simulink model "HEV_powersplit_adapted"  (R2026a)
settings: Solver=VariableStepAuto  StopTime=DriveCycles(Drive_Cycle_Num).time(end)  FixedStep=Ts  AbsTol=1e-3  EnableMultiTasking=on
PreLoadFcn:
  | mdlDir = fileparts(get_param(bdroot,'FileName'));
  | if exist(mdlDir,'dir'), addpath(genpath(mdlDir)); end;
  | HEV_Model_HomeDir = mdlDir;
  | decimation = 1;
  | HEV_Model_PARAM;
  | HEV_SeriesParallel_param_detailed;
StartFcn:
  | tic;
StopFcn:
  | Elapsed_Sim_Time = toc;
undefined symbols (not defined in the file): AH, AH0, Drive_Cycle_Num, HEV_Param, Ld, Lq, p, psim, System, Ts, Vbat, VDC_VECT
libraries: fl_lib x70, nesl_utility x54, ee_lib x10, sdl_lib x6, eeTransforms x4, eePmsmCurrentController x2, eeGeneralControl x2, eePmsmCurrentReferenceGen x2, eePwmGeneratorTwoLevel x2, batteryecm_lib x1, Capacitors_lib x1, eePmsmTorqueEstimator x1
(part 1 of 3)
CloseFcn:
  | try,close(h1_HEV_powersplit_adapted),end
  | try,close(h2_HEV_powersplit_adapted),end
  | try,close(h3_HEV_powersplit_adapted),end
  | try,close(h4_hev_powersplit_adapted_pct),end
  | clear h1_HEV_powersplit_adapted h2_HEV_powersplit_adapted h3_HEV_powersplit_adapted h4_hev_powersplit_adapted_pct
  | clear simlog_HEV_powersplit_adapted logsout_HEV_powersplit_adapted Elapsed_Sim_Time
  | 
  | try,close(h1_IPMSMSeriesParallelHEV),end
  | clear h1_IPMSMSeriesParallelHEV
  | 
  | clear simlog_IPMSMSeriesParallelHEV
  | clear logsout_IPMSMSeriesParallelHEV
  | 
  | clear PmaxEM TmaxEM p psim Ld Lq L0 Rs Jm Cdc Vnom
  | clear Q Vbat Ri AH V1 AH1 SOC0 AH0
  | clear TmaxICE PmaxICE Km Tm
  | clear Ts fsw Tsi Tso Tsd Kp_id Ki_id Kp_iq Ki_iq
  | clear numd_id dend_id numd_iq dend_iq
  | clear Kp_ice Ki_ice Kp_omega Ki_omega numd_omega dend_omega
  | clear ID_MAP IQ_MAP RPM_VECT TQ_VECT VDC_VECT
  | clear Mv g rho_a AL Cd cr1 cr2 Rw ratio i_t
Description:
  | IPMSM Torque Control in a Series-Parallel HEV
  | Copyright 2025 The MathWorks, Inc.
settings Model: NumberOfSteps=100  Creator=The MathWorks, Inc.  LastModifiedBy=gusta
settings DataIOCC: MaxDataPoints=310000  SignalLoggingName=logsout_HEV_powersplit_adapted
settings OptimizationCC: OptimizeBlockIOStorage=off  OptimizeDataStoreBuffers=off  BusAssignmentInplaceUpdate=off
settings DebuggingCC: UnderspecifiedInitializationDetection=Classic  MaxConsecutiveZCsMsg=none  MaskedZcDiagnostic=none  IgnoredZcDiagnostic=none  ParameterPrecisionLossMsg=none
settings RTWCC: GenerateReport=on  BuildConfiguration=Debug  LaunchReport=on
settings CodeAppCC: MATLABSourceComments=on  EnableCustomComments=on
settings GRTTargetCC: MultiInstanceErrorCode=Warning  CombineSignalStateStructs=on  SupportVariableSizeSignals=on
settings SimscapeCC: SimscapeNormalizeSystem=off  SimscapeNominalValues="[{\"value\":\"1\",\"unit\":\"A\"},{\"value\":\"1\",\"unit\":\"bar\"},{\"value\":\"1\",\"unit\":\"cm^2\"},{\"value\":\"1\",\"unit\":\"cm^3/s\"},{\"value\":\"1\",\"unit\":\"kJ/kg\"},{\"value\":\"1\",\"unit\":\"kW\"},{\"value\":\"1\",\"unit\":\"l\"},{\"value\":\"1\",\"unit\":\"N\"},{\"value\":\"1\",\"unit\":\"N*m\"},{\"value\":\"1\",\"unit\":\"V\"}]"  SimscapeLogSimulationStatistics=on  SimscapeLogName=simlog_HEV_powersplit_adapted  SimscapeLogDataHistory=310000.0

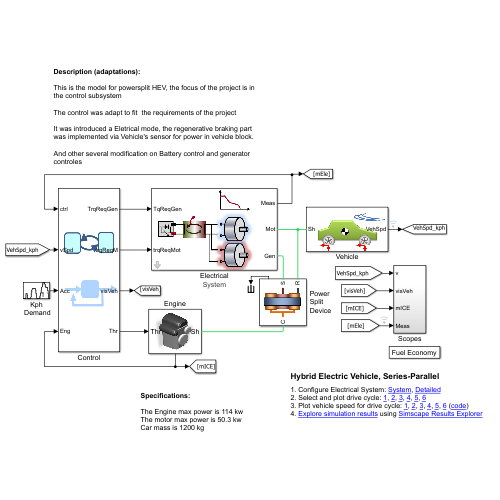
[thumbnail: Simulink's stored preview of the top-level diagram]
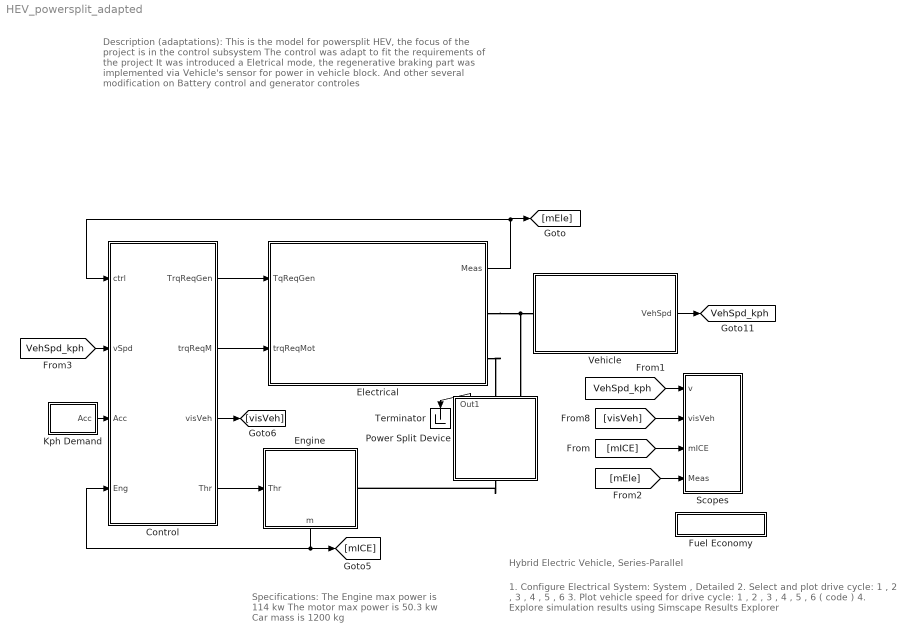
== system HEV_powersplit_adapted ==
  note: Description (adaptations):
      |
      | This is the model for powersplit HEV, the focus of the project is in the control subsystem
      |
      | The control was adapt to fit the requirements of the project
      |
      | It was introduced a Eletrical mode, the regenerative braking part was implemented via Vehicle's sensor for power in vehicle block.
      |
      | And other several modification on Battery control and generator controles
  note: Specifications:
      |
      | The Engine max power is 114 kw
      | The motor max power is 50.3 kw
      | Car mass is 1200 kg
  note: Hybrid Electric Vehicle, Series-Parallel
  note: 1. Configure Electrical System: System , Detailed
      | 2. Select and plot drive cycle: 1 , 2 , 3 , 4 , 5 , 6
      | 3. Plot vehicle speed for drive cycle: 1 , 2 , 3 , 4 , 5 , 6 ( code )
      | 4. Explore simulation results using Simscape Results Explorer
  Control : Subsystem
      mask Display: image('HEV_Control_IMAGE.jpg')
  Electrical : Subsystem  mask{popup_machModelType=System}
      mask prompts: popup_machModelType "Machine Model Type"
      settings: AttributesFormatString=%<popup_machModelType>
      mask TypeOptions popup_machModelType: Generator/popup_modelType | Motor/popup_modelType
      mask Display:
      | bh = gcb;
      | machType = get_param(bh, 'popup_machModelType');
      | if(strcmp(machType,'Detailed'))
      |     image('HEV_Electrical_Detailed_Generic_IMAGE.jpg');
      | else
      |     image('HEV_Electrical_SystemLevel_Generic_IMAGE.jpg');
      | end
  Engine : Subsystem
      settings: PortSchema="{\"entries\":[{\"content\":{\"sides\":[{\"content\":{\"connectorIds\":[\"In1\"]},\"type\":\"ConnectorPlacement.EquallySpacedRectSide\",\"uuid\":\"790115e8-146c-4b4e-bf41-f4d786beb81e\"},{\"content\":{\"connectorIds\":[\"RConn1\"],\"side\":\"RIGHT\"},\"type\":\"ConnectorPlacement.EquallySpacedRectSide\",\"uuid\":\"b4f77556-b395-4615-ac3d-7576af564f11\"},{\"content\":{\"side\":\"TOP\"},\"type\":\"ConnectorPlacement.EquallySpacedRectSide\",\"uuid\":\"44f1e3da-b746-41cb-9fdb-85dae22187d3\"},{\"content\":{\"connectorIds\":[\"Out1\"],\"side\":\"BOTTOM\"},\"type\":\"ConnectorPlacement.EquallySpacedRectSide\",\"uuid\":\"b1d76e0d-1938-4db2-9fd9-287b303ac6ee\"}]},\"type\":\"ConnectorPlacement.EquallySpacedConnector\",\"uuid\":\"a06ee764-44f8-463f-a9be-99a8119a4dd7\"}],\"packageUris\":[\"http://schema.mathworks.com/mf0/Connector/R2020b\"],\"version\":\"1.0\"}"
      mask Display:
      | image('HEV_Engine_IMAGE.jpg');
      | port_label('input',1,'Thr');
      | port_label('RConn',1,'Sh');
  Fuel Economy : Subsystem  mask(Data Acquisition){}
      mask Display: disp('Fuel Economy');
  Kph Demand : Subsystem
      mask Display:
      | %if(evalin('base','Drive_Cycle_Num')<5)
      | plotstr=['UrbanCycle' evalin('base','num2str(Drive_Cycle_Num)')];
      | plot(evalin('base',[plotstr '.time']),evalin('base',[plotstr '.SpdKph']));
      | text(evalin('base',['0.7*max(' plotstr '.time)']),evalin('base',['0.25*max(' plotstr '.SpdKph)']),evalin('base','num2str(Drive_Cycle_Num)'));
      | %end
  Power Split Device : Subsystem
      mask Display:
      | image('HEV_Planetary_Gear_IMAGE.jpg');
      | color('black');
  Scopes : Subsystem
  Terminator : Terminator
  Vehicle : Subsystem  VariantControl=Full
      mask Display: image(imread('HEV_Vehicle_Dynamics_Full_IMAGE.jpg'));
  tag scope: VehSpd_kph=global
  wires:
  Kph Demand/1(Acc) -> Control/3(Acc)
  Control/3(visVeh) -> [visVeh]
  Vehicle/1(VehSpd) -> [VehSpd_kph]
  [visVeh] -> Scopes/2(visVeh)
  [VehSpd_kph] -> Scopes/1(v)
  Control/4(Thr) -> Engine/1(Thr)
  Engine/1(m) -> [mICE], Control/4(Eng)
  Control/1(TrqReqGen) -> Electrical/1(TqReqGen)
  Control/2(trqReqM) -> Electrical/2(trqReqMot)
  Electrical/1(Meas) -> Control/1(ctrl), [mEle]
  [mICE] -> Scopes/3(mICE)
  [mEle] -> Scopes/4(Meas)
  [VehSpd_kph] -> Control/2(vSpd)
  Power Split Device/1(Out1) -> Terminator/1
  connections:
  Electrical/RConn1 -- Power Split Device/RConn2 -- Vehicle/LConn1
  Power Split Device/LConn1 -- Engine/RConn1
  Electrical/RConn2 -- Power Split Device/RConn1

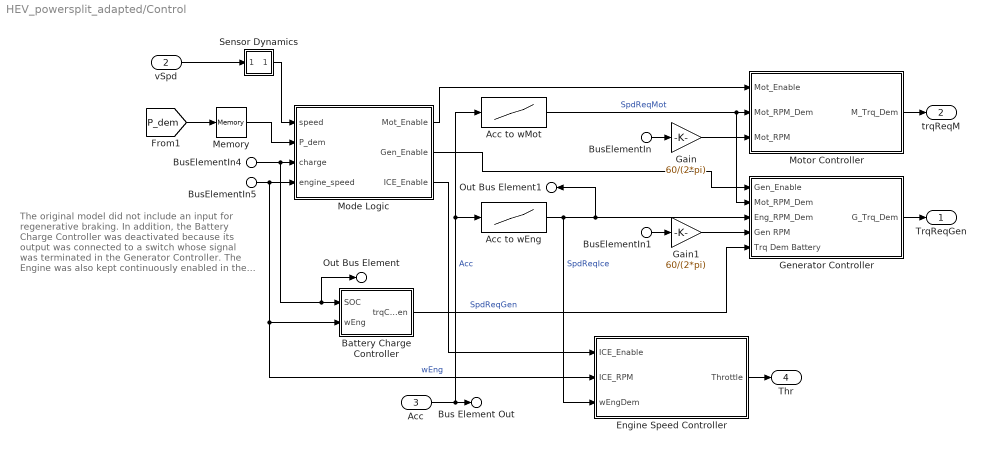
== system HEV_powersplit_adapted/Control ==
  note: The original model did not include an input for regenerative braking. In addition, the Battery Charge Controller was deactivated because its output was connected to a switch whose signal was terminated in the Generator Controller. The Engine was also kept continuously enabled in the Engine Speed Controller, bypassing the mode logic signal.
      | In addition, the sensor signal from the Vehicle block, P_dem , is now used as the power demand input to evaluate all mode transitions, including Regenerative Braking.
  BusElementIn4 : Inport  PortName=ctrl  Element=Batt.SOC
  BusElementIn : Inport  PortName=ctrl  Element=MotCtrl.w
  BusElementIn1 : Inport  PortName=ctrl  Element=GenCtrl.w
  vSpd : Inport  Port=2
  Acc : Inport  Port=3
  BusElementIn5 : Inport  Port=4  PortName=Eng  Element=wEng
  Acc to wEng : Lookup_n-D  NumberOfTableDimensions=1  BreakpointsForDimension1=[0 0.9 0.95 1]  Table=[800 5000 6000 6000]  InternalRulePriority=Speed  RndMeth=Simplest
  Acc to wMot : Lookup_n-D  NumberOfTableDimensions=1  BreakpointsForDimension1=[0 1 1.2]  Table=[0 6000 6000]  InternalRulePriority=Speed  RndMeth=Simplest
  Battery Charge Controller : Subsystem
  Engine Speed Controller : Subsystem
  Gain : Gain  Gain=60/(2*pi)
  Gain1 : Gain  Gain=60/(2*pi)
  Generator Controller : Subsystem
  Memory : Memory
  Mode Logic : Stateflow chart  TreatAsAtomicUnit=on
  Motor Controller : Subsystem
  Sensor Dynamics : Subsystem  mask(First-order lag supporting vector signals){b=HEV_Param.ICE.sensor_time_constant, x_initial=0}
      mask prompts: b "Filter time constant"; x_initial "Initial output"
      mask help: Models a lag of the form 1/(b*s+1) where s is the Laplace operator.
  TrqReqGen : Outport  VectorParamsAs1DForOutWhenUnconnected=off
  trqReqM : Outport  Port=2  VectorParamsAs1DForOutWhenUnconnected=off
  Bus Element Out : Outport  Port=3  PortName=visVeh  Element=Acc
  Out Bus Element : Outport  Port=3  PortName=visVeh  Element=SOC
  Out Bus Element1 : Outport  Port=3  PortName=visVeh  Element=wICEreq
  Thr : Outport  Port=4  VectorParamsAs1DForOutWhenUnconnected=off
  wires:
  Acc/1 -> Acc to wMot/1, Acc to wEng/1, Bus Element Out/1  "Acc"
  Mode Logic/2(Gen_Enable) -> Generator Controller/1(Gen_Enable)
  Generator Controller/1(G_Trq_Dem) -> TrqReqGen/1
  Mode Logic/1(Mot_Enable) -> Motor Controller/1(Mot_Enable)
  BusElementIn/1 -> Gain/1
  Motor Controller/1(M_Trq_Dem) -> trqReqM/1
  Mode Logic/3(ICE_Enable) -> Engine Speed Controller/1(ICE_Enable)
  Engine Speed Controller/1(Throttle) -> Thr/1
  Battery Charge Controller/1(trqCmdGen) -> Generator Controller/5(Trq Dem Battery)  "SpdReqGen"
  Acc to wEng/1 -> Generator Controller/3(Eng_RPM_Dem), Out Bus Element1/1, Engine Speed Controller/3(wEngDem)  "SpdReqIce"
  Acc to wMot/1 -> Generator Controller/2(Mot_RPM_Dem), Motor Controller/2(Mot_RPM_Dem)  "SpdReqMot"
  BusElementIn1/1 -> Gain1/1
  BusElementIn4/1 -> Out Bus Element/1, Battery Charge Controller/1(SOC), Mode Logic/3(charge)
  vSpd/1 -> Sensor Dynamics/1(In)
  BusElementIn5/1 -> Engine Speed Controller/2(ICE_RPM), Battery Charge Controller/2(wEng), Mode Logic/4(engine_speed)  "wEng"
  Sensor Dynamics/1(Out) -> Mode Logic/1(speed)
  Gain/1 -> Motor Controller/3(Mot_RPM)
  Gain1/1 -> Generator Controller/4(Gen RPM)
  [P_dem] -> Memory/1
  Memory/1 -> Mode Logic/2(P_dem)

== system HEV_powersplit_adapted/Electrical ==
  TqReqGen : Inport
  trqReqMot : Inport  Port=2
  DC-DC Converter : Subsystem
      mask Display:
      | patch([-0.9 -1 -1 0.9 1 1 -0.9],[-1 -1 -0.9 1 1 0.9 -1],[0 0 0])
      | 
      | patch([-0.8 -0.1 -0.1 -0.8],[0.85 0.85 0.75 0.75],[0 0 0])
      | patch([-0.8 -0.55 -0.55 -0.8],[0.65 0.65 0.55 0.55],[0 0 0])
      | patch([-0.35 -0.1 -0.1 -0.35],[0.65 0.65 0.55 0.55],[0 0 0])
      | 
      | patch([-0.8 -0.1 -0.1 -0.8]*-1,[0.65 0.65 0.55 0.55]*-1,[0 0 0])
      | patch([-0.8 -0.55 -0.55 -0.8]*-1,[0.85 0.85 0.75 0.75]*-1,[0 0 0])
      | patch([-0.35 -0.1 -0.1 -0.35]*-1,[0.85 0.85 0.75 0.75]*-1,[0 0 0])
  ERef : fl_lib/Electrical/Electrical Elements/Electrical Reference
  Electrical Reference : fl_lib/Electrical/Electrical Elements/Electrical Reference
  Generator : Subsystem  Variant=on  VariantControlMode=label  VariantControl=Generator  LabelModeActiveChoice=System  mask{popup_modelType=System}
      mask prompts: popup_modelType "Model Type"
      mask init:
      | bh = gcb;
      | set_param(bh,'LabelModeActiveChoice',get_param(bh,'popup_modelType'));
      mask TypeOptions popup_modelType: System | Detailed
  Generic : Subsystem  VariantControl=Generic
      mask Display: image('HEV_Battery_Custom_IMAGE.jpg')
  Motor : Subsystem  Variant=on  VariantControlMode=label  VariantControl=Motor  LabelModeActiveChoice=System  mask{popup_modelType=System}
      mask prompts: popup_modelType "Model Type"
      mask init:
      | bh = gcb;
      | set_param(bh,'LabelModeActiveChoice',get_param(bh,'popup_modelType'));
      mask TypeOptions popup_modelType: System | Detailed
  Solver Configuration : nesl_utility/Solver Configuration  PhysicalDomain=network_engine_domain  SubClassName=solver  LeftPortType=input  RightPortType=generic  Tones=[]  Harmonics=[]  SimulateNoise=off  Profile=off  UseLocalSampling=off  EnableSwitchedLinearOptims=on  FrequencyDomain=off  UseCCode=off  RelTol=0.001  AbsTol=1e-06  MinStep=1e-09  ToWorkspace=off  RevertToSquareIcSolve=off  NumHomotopyIterations=100  PhasorMode=off  PhasorModeNumHarmonics=1  ConsistencySolver=NEWTON_FTOL  CanonicalOrdering=UNORDERED  OptimizeIntermediates=UNOPTIMIZED  IndexReductionMethod=DerivativeReplacement  DoDC=off  ResidualTolerance=1e-9  ConsistencyTolSource=GLOBAL  ConsistencyAbsTol=0.001  ConsistencyRelTol=0.001  ConsistencyTolFactor=0.001  UseLocalSolver=off  LocalSolverChoice=NE_BACKWARD_EULER_ADVANCER  ResolveIndetEquations=on  FunctionEvalNumThread=1  LocalSolverSampleTime=Ts  DoFixedCost=off  MaxNonlinIter=4  MaxModeIter=2  ComputeImpulses=off  ImpulseIterations=1  LinearAlgebra=auto  LinearAlgebraNumThread=0  EquationFormulation=NE_TIME_EF  DelaysMemoryBudget=1024  AutomaticFiltering=on  FilteringTimeConstant=0.001  PartitionStorageMethod=AS_NEEDED  PartitionMemoryBudget=1024  PartitionMethod=FAST  MultibodyUseLocalSolver=off  MultibodyLocalSolverChoice=ODE1  MultibodyLocalSolverSampleTime=0.001
  Mot : PMIOPort  Side=Right
  Gen : PMIOPort  Port=2  Side=Right
  Bus Element Out : Outport  PortName=Meas  Element=MotCtrl
  Bus Element Out1 : Outport  PortName=Meas  Element=GenCtrl
  Bus Element Out2 : Outport  PortName=Meas  Element=Batt
  Bus Element Out3 : Outport  PortName=Meas  Element=Gen
  Bus Element Out4 : Outport  PortName=Meas  Element=Mot
  wires:
  trqReqMot/1 -> Motor/1(trqReq)
  Motor/1(meas) -> Bus Element Out4/1
  Motor/2(Ctrl) -> Bus Element Out/1
  TqReqGen/1 -> Generator/1(trqReq)
  Generator/1(meas) -> Bus Element Out3/1
  Generator/2(Ctrl) -> Bus Element Out1/1
  Generic/1(m) -> Bus Element Out2/1
  connections:
  Electrical Reference/LConn1 -- Solver Configuration/RConn1 -- Generic/LConn2 -- DC-DC Converter/LConn2
  Motor/LConn1 -- DC-DC Converter/RConn1 -- Generator/LConn1
  Mot/RConn1 -- Motor/RConn1
  Gen/RConn1 -- Generator/RConn1
  Generator/LConn2 -- Motor/LConn2 -- DC-DC Converter/RConn2 -- ERef/LConn1
  Generic/LConn1 -- DC-DC Converter/LConn1

== system HEV_powersplit_adapted/Engine ==
  Thr : Inport
  Damper : fl_lib/Mechanical/Rotational Elements/Rotational Damper  D=HEV_Param.ICE.Friction N*m/(rad/s)  w_specify=off  w_priority=High  w=0 rad/s  w_nominal_specify=off  w_nominal_value=1  w_nominal_unit=rad/s  t_specify=off  t_priority=High  t=0 N*m  t_nominal_specify=off  t_nominal_value=1  t_nominal_unit=N*m
  Engine Shaft Inertia : fl_lib/Mechanical/Rotational Elements/Inertia  inertia=HEV_Param.ICE.Shaft_Inertia kg*m^2  num_ports=foundation.enum.numPorts2.one  w_specify=on  w_priority=High  w=HEV_Param.Control.Engine_Start_RPM rpm  w_nominal_specify=off  w_nominal_value=1  w_nominal_unit=rad/s  t_specify=off  t_priority=High  t=0 N*m  t_nominal_specify=off  t_nominal_value=1  t_nominal_unit=N*m
  Generic Engine : sdl_lib/Engines & Motors/Generic Engine  input_type=sdl.enum.GenericEngineInputType.NormalizedThrottle  model_parameterization=1  engine_type=1  Trq_max=380 N*m  w_Trq_max=4300 rpm  P_max=HEV_Param.ICE.Max_Power W  w_P_max=HEV_Param.ICE.Speed_At_Max_Power rpm  w_max=HEV_Param.ICE.Max_Speed rpm  w_min=500 rpm  w_tab=[ 500 1000 2e+3 3e+3 4e+3 5e+3 6e+3 7e+3 ] rpm  trq_tab=[ 380 380 380 380 350 280 200 80 ] N*m  pwr_tab=[ 2e+4 4e+4 7.8e+4 1.2e+5 1.45e+5 1.48e+5 1.25e+5 6e+4 ] W  interp_method=1  w_thr=100 rpm  model_inertia=0  inertia=1 kg*m^2  initial_velocity=800 rpm  model_time_constant=0  time_constant=0.2 s  initial_normalized_throttle=0  fc_model=1  fc_per_rev=25 mg/rev  fc_w_tab=[ 1000 2e+3 3e+3 4e+3 5e+3 6e+3 ] rpm  fc_trq_tab=[ 0 80 160 200 240 320 360 400 ] N*m  fc_tab=[ 0.5 0.9 1.4 1.6 1.9 2.7 3.4 4.4; 1 1.7 2.7 3.1 3.6 5 6 7.4; 1.4 2.7 4 4.8 5.6 7.5 8.5 10.5; 2 3.6 5.8 6.7 8 10.4 11.7 13.3; 2.5 4.8 7.9 9.4 10.8 14 16.2 18.6; 3.1 6 10.3 11.9 13.8 18.4 22 26.5 ] g/s  bmep_tab=[ 0 250 500 625 750 1000 1.15e+3 1.25e+3 ] kPa  bsfc_tab=[ 410 380 300 280 270 290 320 380; 410 370 290 270 260 270 285 320; 415 380 290 275 265 270 270 300; 420 390 310 290 285 280 280 285; 430 410 340 320 310 300 310 320; 450 430 370 340 330 330 350 380 ] g/hr/kW  fc_interp_method=1  displaced_volume=400 cm^3  rev_per_cycle=2  idle_speed=0  idle_speed_reference=1000 rpm  tau_controller=1 s  idle_w_thr=1 rpm  redline=0  redline_speed=5000 rpm  tau_redline=1 s  redline_w_thr=1 rpm
  MRRef Engine Housing : fl_lib/Mechanical/Rotational Elements/Mechanical Rotational Reference
  Sensor : Subsystem
      settings: PortSchema="{\"entries\":[{\"content\":{\"sides\":[{\"content\":{\"connectorIds\":[\"LConn1\"]},\"type\":\"ConnectorPlacement.EquallySpacedRectSide\",\"uuid\":\"5a33ac70-cd2c-47ff-b866-bd3f3557f685\"},{\"content\":{\"connectorIds\":[\"RConn1\"],\"side\":\"RIGHT\"},\"type\":\"ConnectorPlacement.EquallySpacedRectSide\",\"uuid\":\"5c843a06-af9b-4ac3-9267-bba109437eb6\"},{\"content\":{\"side\":\"TOP\"},\"type\":\"ConnectorPlacement.EquallySpacedRectSide\",\"uuid\":\"fe58ca13-627c-4f53-907b-1080a8c8494c\"},{\"content\":{\"connectorIds\":[\"Out1\"],\"side\":\"BOTTOM\"},\"type\":\"ConnectorPlacement.EquallySpacedRectSide\",\"uuid\":\"ba14817e-a66b-4663-ba7e-b24568ac9611\"}]},\"type\":\"ConnectorPlacement.EquallySpacedConnector\",\"uuid\":\"5d87e06c-df1a-4ca2-879b-92f90cce612e\"}],\"packageUris\":[\"http://schema.mathworks.com/mf0/Connector/R2020b\"],\"version\":\"1.0\"}"
      mask Display: disp('S');
  Simulink-PS Converter : nesl_utility/Simulink-PS Converter  PhysicalDomain=network_engine_domain  SubClassName=ps_input  LeftPortType=input  RightPortType=output  PseudoPeriodic=off  Frequencies=[]  NoiseDistribution=none  NoiseParameters=[]  Unit=1  AffineConversion=off  FilteringAndDerivatives=zero  SimscapeFilterOrder=1  InputFilterTimeConstant=0.005  UdotUserProvided=0
  Sh : PMIOPort  Side=Right
  m : Outport
  wires:
  Thr/1 -> Simulink-PS Converter/1  "Throttle"
  Sensor/1(m) -> m/1
  connections:
  Simulink-PS Converter/RConn1 -- Generic Engine/LConn1
  MRRef Engine Housing/LConn1 -- Damper/RConn1 -- Generic Engine/LConn2
  Sensor/LConn1 -- Engine Shaft Inertia/LConn1 -- Generic Engine/RConn3 -- Damper/LConn1
  Sh/RConn1 -- Sensor/RConn1

== system HEV_powersplit_adapted/Fuel Economy ==
  note: Fuel Economy
  (L/100 km) : Display
      settings: Decimation=decimation
  (MPG) : Display
      settings: Decimation=decimation
  (km/L) : Display
      settings: Decimation=decimation
  Calculate Fuel Economy : Subsystem
  Fuel Consumption Table : Lookup2D  RowIndex=HEV_Param.ICE.FC.Speed_Vector  ColumnIndex=HEV_Param.ICE.FC.Torque_Vector  Table=HEV_Param.ICE.FC.Consumption_Table  SaturateOnIntegerOverflow=off  InputSameDT=off
  Total Fuel Used (L) : Display
      settings: Decimation=decimation
  wires:
  Calculate Fuel Economy/1(Liter/100Km) -> (L/100 km)/1
  Calculate Fuel Economy/3(MPG) -> (MPG)/1
  [VehSpd_kph] -> Calculate Fuel Economy/1(Kph)
  Calculate Fuel Economy/4(Fuel Used (L)) -> Total Fuel Used (L)/1
  Calculate Fuel Economy/2(Km/Liter) -> (km/L)/1
  Fuel Consumption Table/1 -> Calculate Fuel Economy/2(Fuel Flow g/s)
  [engine_speed] -> Fuel Consumption Table/1
  [Carrier_Trq_Nm] -> Fuel Consumption Table/2

== system HEV_powersplit_adapted/Kph Demand ==
  Drive Cycle 1 : FromWorkspace  VariableName=[DriveCycles(1).time DriveCycles(1).SpdKph]
  Drive Cycle 2 : FromWorkspace  VariableName=[DriveCycles(2).time DriveCycles(2).SpdKph]
  Drive Cycle 3 : FromWorkspace  VariableName=[DriveCycles(3).time DriveCycles(3).SpdKph]
  Drive Cycle 4 : FromWorkspace  VariableName=[DriveCycles(4).time DriveCycles(4).SpdKph]
  Drive Cycle 5 : FromWorkspace  VariableName=[DriveCycles(5).time DriveCycles(5).SpdKph]
  Drive Cycle 6 : FromWorkspace  VariableName=[DriveCycles(6).time DriveCycles(6).SpdKph]
  Multiport Switch : MultiPortSwitch  Inputs=6  SaturateOnIntegerOverflow=off  InputSameDT=off
  Select Cycle : Constant  Value=Drive_Cycle_Num
  Vehicle Speed Controller : Subsystem
  Acc : Outport  VectorParamsAs1DForOutWhenUnconnected=off
  wires:
  Drive Cycle 3/1 -> Multiport Switch/4
  Select Cycle/1 -> Multiport Switch/1
  Drive Cycle 2/1 -> Multiport Switch/3
  Drive Cycle 1/1 -> Multiport Switch/2
  Vehicle Speed Controller/1(Acc) -> Acc/1  "Acc"
  Multiport Switch/1 -> Vehicle Speed Controller/1(Ref Spd)  "RefSpd"
  [VehSpd_kph] -> Vehicle Speed Controller/2(Veh Spd)
  Drive Cycle 4/1 -> Multiport Switch/5
  Drive Cycle 5/1 -> Multiport Switch/6
  Drive Cycle 6/1 -> Multiport Switch/7

== system HEV_powersplit_adapted/Power Split Device ==
  note: Engine
  note: For port placement
  note: Motor & Drivetrain
  note: Generator
  Constant : Constant
  Planetary Gear : sdl_lib/Gears/Planetary Gear  rs_ratio=HEV_Param.Power_Split.Ratio_Ring2Sun  friction_model=2  efficiency=[ 0.96 0.98 ]  temperature_TLU=[ 280 300 320 ] K  efficiency_sp_TLU=[ 0.95 0.9 0.85 ]  efficiency_rp_TLU=[ 0.95 0.9 0.85 ]  pwr_thr=[ 0.001 0.001 ] W  mu_visc=[ 0.02 0 ] N*m/(rad/s)  model_inertia=0  sun_inertia=1e-10 kg*m^2  ring_inertia=1e-10 kg*m^2  carrier_inertia=1e-10 kg*m^2  carrier_radius=0.01 m  planet_inertia=0.001 kg*m^2  planet_mass=1e-10 kg  thermal_mass=50 J/K  T_init=300 K
  Sensor Carrier Shaft : Subsystem
      mask Display: disp('S')
  Sensor Ring Shaft : Subsystem
      mask Display: disp('S')
  Sensor Sun Shaft : Subsystem
      mask Display: disp('S')
  S : PMIOPort  Side=Right
  R : PMIOPort  Port=2  Side=Right
  C : PMIOPort  Port=3  Side=Left
  Out1 : Outport  VectorParamsAs1DForOutWhenUnconnected=off
  wires:
  Constant/1 -> Out1/1
  connections:
  S/RConn1 -- Sensor Sun Shaft/RConn1
  Planetary Gear/RConn1 -- Sensor Ring Shaft/LConn1
  Planetary Gear/RConn2 -- Sensor Sun Shaft/LConn1
  R/RConn1 -- Sensor Ring Shaft/RConn1
  Sensor Carrier Shaft/LConn1 -- C/RConn1
  Sensor Carrier Shaft/RConn1 -- Planetary Gear/LConn1

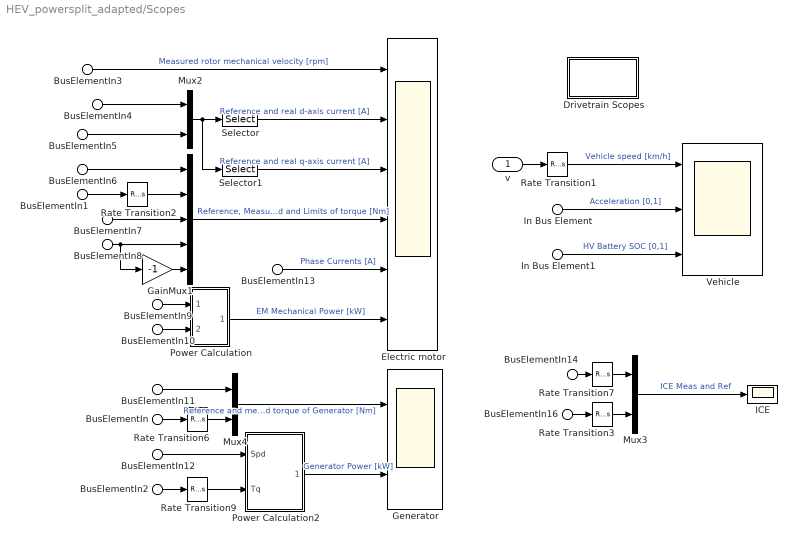
== system HEV_powersplit_adapted/Scopes ==
  v : Inport
  In Bus Element : Inport  Port=2  PortName=visVeh  Element=Acc
  In Bus Element1 : Inport  Port=2  PortName=visVeh  Element=SOC
  BusElementIn14 : Inport  Port=2  PortName=visVeh  Element=wICEreq
  BusElementIn16 : Inport  Port=3  PortName=mICE  Element=wEng
  BusElementIn1 : Inport  Port=4  PortName=Meas  Element=MotCtrl.Tq
  BusElementIn : Inport  Port=4  PortName=Meas  Element=GenCtrl.Tq
  BusElementIn2 : Inport  Port=4  PortName=Meas  Element=GenCtrl.Tq
  BusElementIn3 : Inport  Port=4  PortName=Meas  Element=Mot.Spd
  BusElementIn9 : Inport  Port=4  PortName=Meas  Element=Mot.Spd
  BusElementIn4 : Inport  Port=4  PortName=Meas  Element=Mot.idqRef
  BusElementIn5 : Inport  Port=4  PortName=Meas  Element=Mot.idq
  BusElementIn6 : Inport  Port=4  PortName=Meas  Element=Mot.TqRef
  BusElementIn7 : Inport  Port=4  PortName=Meas  Element=Mot.TqEstim
  BusElementIn10 : Inport  Port=4  PortName=Meas  Element=Mot.TqEstim
  BusElementIn8 : Inport  Port=4  PortName=Meas  Element=Mot.TqLim
  BusElementIn13 : Inport  Port=4  PortName=Meas  Element=Mot.iabc
  BusElementIn11 : Inport  Port=4  PortName=Meas  Element=Gen.TqRef
  BusElementIn12 : Inport  Port=4  PortName=Meas  Element=Gen.Spd
  Drivetrain Scopes : Subsystem
  Electric motor : Scope  NumInputPorts=6
      settings: ActiveDisplayYMinimum=-2.81918  ActiveDisplayYMaximum=25.3726
  Gain : Gain  Gain=-1
  Generator : Scope  NumInputPorts=2
      settings: ActiveDisplayYMinimum=-96.70372  ActiveDisplayYMaximum=183.60525  DataLoggingVariableName=ScopeData2
  ICE : Scope
      settings: ActiveDisplayYMinimum=788.66371773526942  ActiveDisplayYMaximum=802.79610145254
  Mux1 : Mux  Inputs=5
  Mux2 : Mux  Inputs=2
  Mux3 : Mux  Inputs=2
  Mux4 : Mux  Inputs=2
  Power Calculation2 : Subsystem
  Power Calculation : Subsystem
  Rate Transition{1..3,6..7,9} (6 alike) : RateTransition
  Selector : Selector  InputPortWidth=4  IndexOptions=Index vector (dialog)  Indices=[1 3]  OutputSizes=1
  Selector1 : Selector  InputPortWidth=4  IndexOptions=Index vector (dialog)  Indices=[2 4]  OutputSizes=1
  Vehicle : Scope  NumInputPorts=3
      settings: ActiveDisplayYMinimum=0.29062931672559955  ActiveDisplayYMaximum=56.824123356677326
  wires:
  BusElementIn3/1 -> Electric motor/1  "Measured rotor mechanical velocity [rpm]"
  BusElementIn6/1 -> Mux1/1
  BusElementIn8/1 -> Mux1/4, Gain/1
  v/1 -> Rate Transition1/1
  In Bus Element/1 -> Vehicle/2  "Acceleration [0,1]"
  BusElementIn4/1 -> Mux2/1
  Mux2/1 -> Selector1/1, Selector/1
  BusElementIn5/1 -> Mux2/2
  BusElementIn1/1 -> Rate Transition2/1
  Gain/1 -> Mux1/5
  Rate Transition2/1 -> Mux1/2
  BusElementIn7/1 -> Mux1/3
  BusElementIn9/1 -> Power Calculation/1(Spd)
  BusElementIn10/1 -> Power Calculation/2(Tq)
  Mux3/1 -> ICE/1  "ICE Meas and Ref"
  BusElementIn16/1 -> Rate Transition3/1
  In Bus Element1/1 -> Vehicle/3  "HV Battery SOC [0,1]"
  BusElementIn2/1 -> Rate Transition9/1
  Power Calculation2/1(Power) -> Generator/2  "Generator Power [kW]"
  BusElementIn/1 -> Rate Transition6/1
  BusElementIn11/1 -> Mux4/1
  Mux4/1 -> Generator/1  "Reference and measured torque of Generator [Nm]"
  Rate Transition3/1 -> Mux3/2
  Rate Transition7/1 -> Mux3/1
  Rate Transition9/1 -> Power Calculation2/2(Tq)
  Rate Transition6/1 -> Mux4/2
  BusElementIn12/1 -> Power Calculation2/1(Spd)
  BusElementIn14/1 -> Rate Transition7/1
  Mux1/1 -> Electric motor/4  "Reference, Measured,Estimated and Limits of torque [Nm]"
  Selector/1 -> Electric motor/2  "Reference and real d-axis current [A]"
  Selector1/1 -> Electric motor/3  "Reference and real q-axis current [A]"
  BusElementIn13/1 -> Electric motor/5  "Phase Currents [A]"
  Power Calculation/1(Power) -> Electric motor/6  "EM Mechanical Power [kW]"
  Rate Transition1/1 -> Vehicle/1  "Vehicle speed [km/h]"

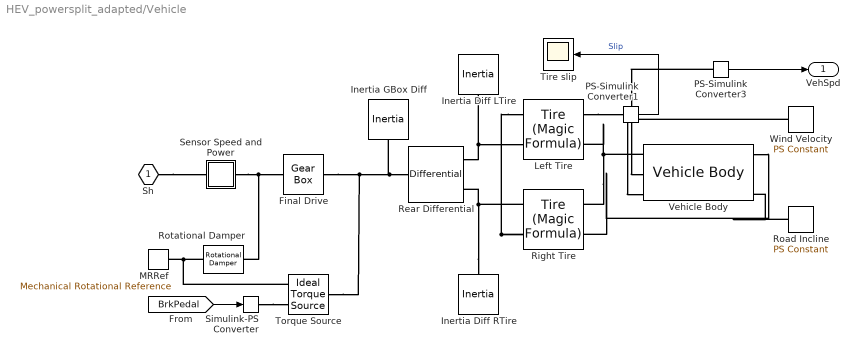
== system HEV_powersplit_adapted/Vehicle ==
  Final Drive : fl_lib/Mechanical/Mechanisms/Gear Box  ratio=HEV_Param.Vehicle.Engine_Vehicle_Gear_Ratio  t_in_specify=off  t_in_priority=None  t_in=0 N*m  t_in_nominal_specify=off  t_in_nominal_value=1  t_in_nominal_unit=N*m  t_out_specify=off  t_out_priority=None  t_out=0 N*m  t_out_nominal_specify=off  t_out_nominal_value=1  t_out_nominal_unit=N*m
  Inertia Diff LTire : fl_lib/Mechanical/Rotational Elements/Inertia  inertia=HEV_Param.Vehicle.Wheel_Inertia*2 kg*m^2  num_ports=foundation.enum.numPorts2.one  w_specify=on  w_priority=High  w=0 rad/s  w_nominal_specify=off  w_nominal_value=1  w_nominal_unit=rad/s  t_specify=off  t_priority=High  t=0 N*m  t_nominal_specify=off  t_nominal_value=1  t_nominal_unit=N*m
  Inertia Diff RTire : fl_lib/Mechanical/Rotational Elements/Inertia  inertia=HEV_Param.Vehicle.Wheel_Inertia*2 kg*m^2  num_ports=foundation.enum.numPorts2.one  w_specify=on  w_priority=High  w=0 rad/s  w_nominal_specify=off  w_nominal_value=1  w_nominal_unit=rad/s  t_specify=off  t_priority=High  t=0 N*m  t_nominal_specify=off  t_nominal_value=1  t_nominal_unit=N*m
  Inertia GBox Diff : fl_lib/Mechanical/Rotational Elements/Inertia  inertia=HEV_Param.Vehicle.Trans.Inertia kg*m^2  num_ports=foundation.enum.numPorts2.one  w_specify=on  w_priority=High  w=0 rad/s  w_nominal_specify=off  w_nominal_value=1  w_nominal_unit=rad/s  t_specify=off  t_priority=High  t=0 N*m  t_nominal_specify=off  t_nominal_value=1  t_nominal_unit=N*m
  Left Tire : sdl_lib/Tires & Vehicles/Tire (Magic Formula)  parameterization=1  F_z1=HEV_Param.Vehicle.Tire.Rated_Vertical_Load N  F_x1=HEV_Param.Vehicle.Tire.Rated_Peak_Long_Force N  kappa1=HEV_Param.Vehicle.Tire.Slip_At_Peak_Force  B_m=10  C_m=1.9  D_m=1  E_m=0.97  fz0=4e+3 N  p_Cx=1.685  p_Dx=[ 1.21 -0.037 ]  p_Ex=[ 0.344 0.095 -0.02 0 ]  p_Kx=[ 21.51 -0.163 0.245 ]  p_Hx=[ -0.002 0.002 ]  p_Vx=[ 0 0 ]  rolling_radius_model=sdl.enum.RollingRadiusParameterization.Constant  r_e=HEV_Param.Vehicle.Tire_Radius m  r_0=0.3 m  breff=8.39  dreff=0.26  freff=0.074  q_re0=0.99  q_v1=0.008  longvl=17 m/s  cz=5e5 N/m  model_resistance=0  resistance_model=1  coeff=0.015  p_tire=250e3 Pa  alpha=-0.003  beta=0.97  coeff_a=84e-4  coeff_b=6.2e-4 s/m  coeff_c=1.6e-4 s^2/m^2  p_tire0=240e3 Pa  fz0_resistance=4000 N  vH0=16 m/s  q_Sy=[.0082, 0, .0014, .001, 0, 0, 1.08, -.5]  v_thr=1e-3 m/s  enable_scaling_coefficients=false  lfzO=1  lcx=1  lmux=1  lex=1  lkx=1  lhx=1  lvx=1  lmy=1  model_compliance=0  stiffness=1e+6 N/m  damping=1000 N/(m/s)  model_inertia=1  inertia=1e-2 kg*m^2  initial_velocity=0 rpm  vxlow=0.1 m/s  v_tr_thr=0.1*(0.1) m/s  kpumin=-1e5  kpumax=1e5
  MRRef : fl_lib/Mechanical/Rotational Elements/Mechanical Rotational Reference
  PS-Simulink Converter1 : nesl_utility/PS-Simulink Converter  PhysicalDomain=network_engine_domain  SubClassName=ps_output  LeftPortType=input  RightPortType=output  PseudoPeriodic=off  Frequencies=[]  VectorFormat=1-D array  Unit=1  AffineConversion=off
  PS-Simulink Converter3 : nesl_utility/PS-Simulink Converter  PhysicalDomain=network_engine_domain  SubClassName=ps_output  LeftPortType=input  RightPortType=output  PseudoPeriodic=off  Frequencies=[]  VectorFormat=1-D array  Unit=km/hr  AffineConversion=off
  Rear Differential : sdl_lib/Gears/Differential  driveshaft_location=2  cd_ratio=1  friction_model=1  efficiency=[ 0.85 0.92 ]  temperature_TLU=[ 280 300 320 ] K  efficiency_ss_TLU=[ 0.95 0.9 0.85 ]  efficiency_cd_TLU=[ 0.95 0.9 0.85 ]  pwr_thr=[ 0.001 0.001 ] W  mu_visc=[ 0 0 ] N*m/(rad/s)  model_inertia=0  sun_inertia=1e-10 kg*m^2  sun_radius=0.01 m  carrier_inertia=0.001 kg*m^2  planet_inertia=0.001 kg*m^2  planet_mass=1e-10 kg  thermal_mass=50 J/K  T_init=300 K
  Right Tire : sdl_lib/Tires & Vehicles/Tire (Magic Formula)  parameterization=1  F_z1=HEV_Param.Vehicle.Tire.Rated_Vertical_Load N  F_x1=HEV_Param.Vehicle.Tire.Rated_Peak_Long_Force N  kappa1=HEV_Param.Vehicle.Tire.Slip_At_Peak_Force  B_m=10  C_m=1.9  D_m=1  E_m=0.97  fz0=4e+3 N  p_Cx=1.685  p_Dx=[ 1.21 -0.037 ]  p_Ex=[ 0.344 0.095 -0.02 0 ]  p_Kx=[ 21.51 -0.163 0.245 ]  p_Hx=[ -0.002 0.002 ]  p_Vx=[ 0 0 ]  rolling_radius_model=sdl.enum.RollingRadiusParameterization.Constant  r_e=HEV_Param.Vehicle.Tire_Radius m  r_0=0.3 m  breff=8.39  dreff=0.26  freff=0.074  q_re0=0.99  q_v1=0.008  longvl=17 m/s  cz=5e5 N/m  model_resistance=0  resistance_model=1  coeff=0.015  p_tire=250e3 Pa  alpha=-0.003  beta=0.97  coeff_a=84e-4  coeff_b=6.2e-4 s/m  coeff_c=1.6e-4 s^2/m^2  p_tire0=240e3 Pa  fz0_resistance=4000 N  vH0=16 m/s  q_Sy=[.0082, 0, .0014, .001, 0, 0, 1.08, -.5]  v_thr=1e-3 m/s  enable_scaling_coefficients=false  lfzO=1  lcx=1  lmux=1  lex=1  lkx=1  lhx=1  lvx=1  lmy=1  model_compliance=0  stiffness=1e+6 N/m  damping=1000 N/(m/s)  model_inertia=1  inertia=1e-2 kg*m^2  initial_velocity=0 rpm  vxlow=0.1 m/s  v_tr_thr=0.1*(0.1) m/s  kpumin=-1e5  kpumax=1e5
  Road Incline : fl_lib/Physical Signals/Sources/PS Constant  constant=HEV_Param.Vehicle.Incline
  Rotational Damper : fl_lib/Mechanical/Rotational Elements/Rotational Damper  D=HEV_Param.Vehicle.Trans.Friction N*m/(rad/s)  w_specify=off  w_priority=High  w=0 rad/s  w_nominal_specify=off  w_nominal_value=1  w_nominal_unit=rad/s  t_specify=off  t_priority=High  t=0 N*m  t_nominal_specify=off  t_nominal_value=1  t_nominal_unit=N*m
  Sensor Speed and Power : Subsystem
      mask Display: disp('S')
  Simulink-PS Converter : nesl_utility/Simulink-PS Converter  PhysicalDomain=network_engine_domain  SubClassName=ps_input  LeftPortType=input  RightPortType=output  PseudoPeriodic=off  Frequencies=[]  NoiseDistribution=none  NoiseParameters=[]  Unit=1  AffineConversion=off  FilteringAndDerivatives=filter  SimscapeFilterOrder=1  InputFilterTimeConstant=0.05  UdotUserProvided=0
  Tire slip : Scope
      settings: ActiveDisplayYMinimum=-0.00683  ActiveDisplayYMaximum=0.00972  DataLoggingMaxPoints=500000
  Torque Source : fl_lib/Mechanical/Mechanical Sources/Ideal Torque Source
  Vehicle Body : sdl_lib/Tires & Vehicles/Vehicle Body  mass=HEV_Param.Vehicle.Mass kg  n_w=2  x_f=HEV_Param.Vehicle.Distance_CG_FrontAxle m  x_r=HEV_Param.Vehicle.Distance_CG_RearAxle m  y_c=HEV_Param.Vehicle.Distance_CG_Ground m  mass_var=simscape.enum.onoff.off  g=9.81 m/s^2  liftoff_warning=0  area=HEV_Param.Vehicle.Frontal_Area m^2  Cd_var=false  Cd=HEV_Param.Vehicle.Aero_Drag_Coeff  rho=1.18 kg/m^3  model_pitch=0  inertia=4000 kg*m^2  suspension_model=1  k_f=1e4 N/m  b_f=1e4 N/(m/s)  k_r=1e4 N/m  b_r=1e4 N/(m/s)  k_f_TLU=[-2000, -1000, 0, 1000, 2000] N  x_f_TLU=[-.4, -.2, 0, .2, .4] m  b_f_TLU=[-200, -100, 0, 100, 200] N  v_f_TLU=[-4, -2, 0, 2, 4] m/s  k_r_TLU=[-2000, -1000, 0, 1000, 2000] N  x_r_TLU=[-.4, -.2, 0, .2, .4] m  b_r_TLU=[-200, -100, 0, 100, 200] N  v_r_TLU=[-4, -2, 0, 2, 4] m/s  interp_method=simscape.enum.interpolation.linear  extrap_method=simscape.enum.extrapolation.linear  model_hardstop=0  upper_bound_f=.25 m  lower_bound_f=-.25 m  stop_k_f=1e6 N/m  stop_b_f=150 N/(m/s)  upper_bound_r=.25 m  lower_bound_r=-.25 m  stop_k_r=1e6 N/m  stop_b_r=150 N/(m/s)  initial_pitch=0 rad  initial_pitch_rate=0 rad/s  v_specify=on  v_priority=High  v=0 m/s  v_nominal_specify=off  v_nominal_value=1  v_nominal_unit=m/s
  Wind Velocity : fl_lib/Physical Signals/Sources/PS Constant  constant=0
  Sh : PMIOPort  Side=Left
  VehSpd : Outport  VectorParamsAs1DForOutWhenUnconnected=off
  wires:
  [BrkPedal] -> Simulink-PS Converter/1
  PS-Simulink Converter1/1 -> Tire slip/1  "Slip"
  PS-Simulink Converter3/1 -> VehSpd/1
  connections:
  Simulink-PS Converter/RConn1 -- Torque Source/RConn1
  MRRef/LConn1 -- Torque Source/RConn2 -- Rotational Damper/RConn1
  Rotational Damper/LConn1 -- Final Drive/LConn1 -- Sensor Speed and Power/RConn1
  Inertia Diff RTire/LConn1 -- Rear Differential/RConn1 -- Right Tire/LConn2
  Inertia Diff LTire/LConn1 -- Left Tire/LConn2 -- Rear Differential/RConn2
  Left Tire/RConn1 -- PS-Simulink Converter1/LConn1
  PS-Simulink Converter3/LConn1 -- Vehicle Body/LConn2
  Wind Velocity/RConn1 -- Vehicle Body/LConn3
  Road Incline/RConn1 -- Vehicle Body/RConn3
  Left Tire/LConn1 -- Right Tire/LConn1 -- Vehicle Body/RConn1
  Vehicle Body/LConn1 -- Right Tire/RConn2 -- Left Tire/RConn2
  Sh/RConn1 -- Sensor Speed and Power/LConn1
  Final Drive/RConn1 -- Inertia GBox Diff/LConn1 -- Rear Differential/LConn1 -- Torque Source/LConn1

== system HEV_powersplit_adapted/Control/Battery Charge Controller ==
  SOC : Inport
  wEng : Inport  Port=2
  20% torque alowed to charge the battery : Gain  Gain=-0.2
  Constant1 : Constant  Value=0  SampleTime=-1
  Engine-Generator Gear Ratio : Gain  Gain=1/2
  ICE_Characteristics : Lookup_n-D  NumberOfTableDimensions=1  BreakpointsForDimension1=[1000 1500 1800 2000 2500 3000 3800 4500]  Table=[140 180 210 230 250 245 230 200]  InternalRulePriority=Speed  RndMeth=Simplest
  No charging when state of charge greather than 80% : Switch  Threshold=0.8  ZeroCross=off  SaturateOnIntegerOverflow=off  InputSameDT=off
  trqCmdGen : Outport
  wires:
  20% torque alowed to charge the battery/1 -> No charging when state of charge greather than 80%/3
  Constant1/1 -> No charging when state of charge greather than 80%/1
  ICE_Characteristics/1 -> Engine-Generator Gear Ratio/1
  Engine-Generator Gear Ratio/1 -> 20% torque alowed to charge the battery/1
  No charging when state of charge greather than 80%/1 -> trqCmdGen/1
  SOC/1 -> No charging when state of charge greather than 80%/2
  wEng/1 -> ICE_Characteristics/1

== system HEV_powersplit_adapted/Control/Engine Speed Controller ==
  note: Engine speed controller. For demands below the idle speed of
      | 800 rpm the speed demand is set to zero.
  ICE_Enable : Inport
  ICE_RPM : Inport  Port=2
  wEngDem : Inport  Port=3
  20Hz Lowpass Filter : TransferFcn  Denominator=[1/(2*pi*20) 1]
  Engine Idle : Constant  Value=0
  Engine Running : Subsystem
  Ki : Gain  Gain=HEV_Param.Control.ICE.Ki
  Kp : Gain  Gain=HEV_Param.Control.ICE.Kp
  Limits [0,1] : Integrator  ExternalReset=either  LimitOutput=on  UpperSaturationLimit=1  LowerSaturationLimit=0
  Sum : Sum  Inputs=-+|
  Sum1 : Sum  Inputs=++|
  Switch : Switch  Threshold=0.5  ZeroCross=off  SaturateOnIntegerOverflow=off  InputSameDT=off
  "[0,1]" : Saturate  UpperLimit=1  LowerLimit=0
  Throttle : Outport  VectorParamsAs1DForOutWhenUnconnected=off
  wires:
  ICE_RPM/1 -> 20Hz Lowpass Filter/1
  Sum/1 -> Ki/1, Kp/1
  Ki/1 -> Limits [0,1]/1
  Kp/1 -> Sum1/2
  Limits [0,1]/1 -> Sum1/1
  20Hz Lowpass Filter/1 -> Sum/1
  wEngDem/1 -> Switch/1
  "[0,1]"/1 -> Throttle/1
  Sum1/1 -> "[0,1]"/1
  Engine Idle/1 -> Switch/3
  ICE_Enable/1 -> Engine Running/1(ICE_Enable)
  Engine Running/1(Engine Running) -> Switch/2, Limits [0,1]/2
  Switch/1 -> Sum/2

== system HEV_powersplit_adapted/Control/Generator Controller ==
  note: Alternate logic if engine
      | can be turned off
  Gen_Enable : Inport
  Mot_RPM_Dem : Inport  Port=2
  Eng_RPM_Dem : Inport  Port=3
  Gen RPM : Inport  Port=4
  Trq Dem Battery : Inport  Port=5
  Enable Torque Demand : Subsystem
  Mux1 : Mux  Inputs=2
  Set generator RPM so that engine RPM is controlled to zero or the idle speed : Fcn  Expr=(1+HEV_Param.Power_Split.Ratio_Ring2Sun)*u(2)-HEV_Param.Power_Split.Ratio_Ring2Sun*u(1)
  Speed controller : Subsystem
  Subsystem1 : Subsystem
      mask Display: disp('S')
  Torque or Speed Control : Switch  Threshold=0.5  ZeroCross=off  SaturateOnIntegerOverflow=off  InputSameDT=off
  G_Trq_Dem : Outport  VectorParamsAs1DForOutWhenUnconnected=off
  wires:
  Set generator RPM so that engine RPM is controlled to zero or the idle speed/1 -> Subsystem1/1(In1)
  Mux1/1 -> Set generator RPM so that engine RPM is controlled to zero or the idle speed/1
  Gen RPM/1 -> Speed controller/2(W)
  Subsystem1/1(Gen_RPM_Dem) -> Speed controller/1(Wref)
  Trq Dem Battery/1 -> Torque or Speed Control/1
  Gen_Enable/1 -> Enable Torque Demand/1(Gen_Enable)
  [engine_running] -> Torque or Speed Control/2
  Eng_RPM_Dem/1 -> Mux1/2  "Eng RPM Dem"
  Enable Torque Demand/1(G_Trq_Dem) -> G_Trq_Dem/1  "Gen Trq Dem"
  Mot_RPM_Dem/1 -> Mux1/1  "Mot RPM Dem"
  Speed controller/1(Tref) -> Torque or Speed Control/3
  Torque or Speed Control/1 -> Enable Torque Demand/2(TrqDemCtrl)

== system HEV_powersplit_adapted/Control/Motor Controller ==
  note: This loop controls motor speed. The maximum value for V_wref is 5 volts.
  Mot_Enable : Inport
  Mot_RPM_Dem : Inport  Port=2
  Mot_RPM : Inport  Port=3
  20Hz Lowpass Filter : TransferFcn  Denominator=[1/(2*pi*20) 1]
  Enable Torque Demand : Subsystem
  Ki : Gain  Gain=HEV_Param.Control.Mot.Ki
  Kp : Gain  Gain=HEV_Param.Control.Mot.Kp
  Limits [-5,5] : Integrator  LimitOutput=on  UpperSaturationLimit=5  LowerSaturationLimit=-5
  Mot RPM to V : Gain  Gain=5/6700
  Sum : Sum  Inputs=-+|
  Sum1 : Sum  Inputs=++|
  Volts/Nm : Gain  Gain=400/5
  "[-5,5]" : Saturate  UpperLimit=5  LowerLimit=-5
  rpm2volts : Gain  Gain=5/6500
  M_Trq_Dem : Outport  VectorParamsAs1DForOutWhenUnconnected=off
  wires:
  "[-5,5]"/1 -> Volts/Nm/1
  Mot_RPM/1 -> Mot RPM to V/1
  Sum1/1 -> "[-5,5]"/1
  Sum/1 -> Ki/1, Kp/1
  Ki/1 -> Limits [-5,5]/1
  Kp/1 -> Sum1/2
  Limits [-5,5]/1 -> Sum1/1
  20Hz Lowpass Filter/1 -> Sum/1
  rpm2volts/1 -> Sum/2
  Mot RPM to V/1 -> 20Hz Lowpass Filter/1
  Volts/Nm/1 -> Enable Torque Demand/2(TrqDemCtrl)
  Mot_RPM_Dem/1 -> rpm2volts/1
  Mot_Enable/1 -> Enable Torque Demand/1(Mot_Enable)
  Enable Torque Demand/1(TrqDem) -> M_Trq_Dem/1

== system HEV_powersplit_adapted/Control/Sensor Dynamics ==
  In : Inport
  Gain : Gain  Gain=1/b
  Integrator : Integrator  InitialCondition=x_initial
  Sum : Sum  Inputs=|+-  InputSameDT=on  SaturateOnIntegerOverflow=on  OutDataTypeStr=Inherit: Same as first input
  Out : Outport  VectorParamsAs1DForOutWhenUnconnected=off
  wires:
  Sum/1 -> Integrator/1
  In/1 -> Sum/1
  Integrator/1 -> Gain/1
  Gain/1 -> Sum/2, Out/1

== system HEV_powersplit_adapted/Electrical/DC-DC Converter ==
  Ideal Transformer : fl_lib/Electrical/Electrical Elements/Ideal Transformer  n=1/1.4  i1_specify=off  i1_priority=None  i1=0 A  i1_nominal_specify=off  i1_nominal_value=1  i1_nominal_unit=A  v1_specify=off  v1_priority=None  v1=0 V  v1_nominal_specify=off  v1_nominal_value=1  v1_nominal_unit=V  i2_specify=off  i2_priority=None  i2=0 A  i2_nominal_specify=off  i2_nominal_value=1  i2_nominal_unit=A  v2_specify=off  v2_priority=None  v2=0 V  v2_nominal_specify=off  v2_nominal_value=1  v2_nominal_unit=V
  2+ : PMIOPort  Side=Right
  1+ : PMIOPort  Port=2  Side=Left
  1- : PMIOPort  Port=3  Side=Left
  2- : PMIOPort  Port=4  Side=Right
  connections:
  Ideal Transformer/LConn1 -- 1+/RConn1
  Ideal Transformer/RConn1 -- 2+/RConn1
  Ideal Transformer/RConn2 -- 2-/RConn1
  Ideal Transformer/LConn2 -- 1-/RConn1

== system HEV_powersplit_adapted/Electrical/Generator ==
  trqReq : Inport
  Detailed : Subsystem  VariantControl=Detailed
      mask Display: image('HEV_Detailed_Generator_IMAGE.jpg')
  System : Subsystem  VariantControl=System
      mask Display: image('HEV_System_Generator_IMAGE.jpg')
  + : PMIOPort  Side=Left
  R : PMIOPort  Port=2  Side=Right
  - : PMIOPort  Port=3  Side=Left
  meas : Outport
  Ctrl : Outport  Port=2

== system HEV_powersplit_adapted/Electrical/Generic ==
  " Battery" : batteryecm_lib/Battery  Vnom=Vbat V  prm_dir=1  R1_dis=2 Ohm  R1_ch=2 Ohm  R1=Ri Ohm  prm_AH=simscape.enum.battery.prm_AH.finite  AH=AH hr*A  V1=V1 V  AH1=AH1 hr*A  prm_R2=1  R2=inf Ohm  Tmeas=298.15 K  charge_measurement_port=simscape.enum.battery.enable.no  prm_dyn=1  Rp1=0.005 Ohm  tau1=30 s  Rp2=0.005 Ohm  tau2=30 s  Rp3=0.005 Ohm  tau3=30 s  Rp4=0.005 Ohm  tau4=30 s  Rp5=0.005 Ohm  tau5=30 s  prm_fade=1  N_fade=100  AH_fade=45 hr*A  R1_fade=2.02 Ohm  R1_ch_fade=2.02 Ohm  V1_fade=10.35 V  prm_age=1  prm_age_OCV=1  OCV_age=0.9  SOC_age=60  Tmeas_age=298.15 K  delta_time_age_vec=[0] d  temperature_age_vec=[273] K  OCV_scaling_age=2.2134e6  OCV_offset_age=1.632e6  temp_exp_age=0.515833569 V  t_exp_age=0.75  Vnom_T2=12 V  R1_T2=2.2 Ohm  R1_T2_dis=2.2 Ohm  R1_T2_ch=2.2 Ohm  V1_T2=11.4 V  R2_T2=2200 Ohm  Rp1_T2=0.005 Ohm  tau1_T2=30 s  Rp2_T2=0.005 Ohm  tau2_T2=30 s  Rp3_T2=0.005 Ohm  tau3_T2=30 s  Rp4_T2=0.005 Ohm  tau4_T2=30 s  Rp5_T2=0.005 Ohm  tau5_T2=30 s  Tmeas2=273.15 K  thermal_port=simscape.enum.thermaleffects.omit  thermal_mass=30000 J/K  i_specify=off  i_priority=None  i=0 A  i_nominal_specify=off  i_nominal_value=1  i_nominal_unit=A  v_specify=off  v_priority=None  v=0 V  v_nominal_specify=off  v_nominal_value=1  v_nominal_unit=V  charge_specify=on  charge_priority=High  charge=AH0 hr*A  charge_nominal_specify=off  charge_nominal_value=1  charge_nominal_unit=A*hr  num_cycles_specify=off  num_cycles_priority=High  num_cycles=0  num_cycles_nominal_specify=off  num_cycles_nominal_value=1  num_cycles_nominal_unit=1  temperature_specify=off  temperature_priority=High  temperature=298.15 K  temperature_nominal_specify=off  temperature_nominal_value=1  temperature_nominal_unit=K
  Current Sensor : fl_lib/Electrical/Electrical Sensors/Current Sensor
  Lossy Ultracapacitor : Capacitors_lib/Lossy Ultracapacitor  C0=HEV_Param.UltraCapacitor.Nominal_Capacitance F  Cv=HEV_Param.UltraCapacitor.Rate_C_V F/V  R=HEV_Param.UltraCapacitor.Series_R Ohm  Rd=HEV_Param.UltraCapacitor.Self_Discharge_R Ohm  i_specify=off  i_priority=High  i=0 A  i_nominal_specify=off  i_nominal_value=1  i_nominal_unit=A  vc_specify=off  vc_priority=High  vc=0 V  vc_nominal_specify=off  vc_nominal_value=1  vc_nominal_unit=V
  Measurements1 : Subsystem
  Terminator : Terminator
  Terminator1 : Terminator
  Voltage Sensor : fl_lib/Electrical/Electrical Sensors/Voltage Sensor
  + : PMIOPort  Side=Left
  - : PMIOPort  Port=2  Side=Left
  Bus Element Out : Outport  PortName=m  Element=SOC
  wires:
  Measurements1/1(Batt_Ah) -> Terminator/1
  Measurements1/2(Batt_Meas) -> Terminator1/1
  Measurements1/3(SOC) -> Bus Element Out/1
  connections:
  +/RConn1 -- Voltage Sensor/LConn1 -- " Battery"/LConn1 -- Lossy Ultracapacitor/LConn1
  Current Sensor/RConn2 -- Voltage Sensor/RConn2 -- " Battery"/RConn1 -- Lossy Ultracapacitor/RConn1
  -/RConn1 -- Current Sensor/LConn1
  Measurements1/LConn1 -- Voltage Sensor/RConn1
  Current Sensor/RConn1 -- Measurements1/LConn2

== system HEV_powersplit_adapted/Electrical/Motor ==
  trqReq : Inport
  Detailed : Subsystem  VariantControl=Detailed
      mask Display: image('HEV_Detailed_Motor_IMAGE.jpg')
  System : Subsystem  VariantControl=System
      mask Display: image('HEV_System_Motor_IMAGE.jpg')
  + : PMIOPort  Side=Left
  R : PMIOPort  Port=2  Side=Right
  - : PMIOPort  Port=3  Side=Left
  meas : Outport
  Ctrl : Outport  Port=2

== system HEV_powersplit_adapted/Engine/Sensor ==
  Bus Creator : BusCreator  Inputs=3
  Ideal Rotational Motion Sensor : fl_lib/Mechanical/Mechanical Sensors/Ideal Rotational Motion Sensor  reference=foundation.enum.MeasurementReference.difference  acceleration_port=false  velocity_port=true  position_port=true  wrap_angle=simscape.enum.onoff.off  offset=0 rad
  Ideal Torque Sensor : fl_lib/Mechanical/Mechanical Sensors/Ideal Torque Sensor
  Mechanical Rotational Reference : fl_lib/Mechanical/Rotational Elements/Mechanical Rotational Reference
  PS-Simulink Converter : nesl_utility/PS-Simulink Converter  PhysicalDomain=network_engine_domain  SubClassName=ps_output  LeftPortType=input  RightPortType=output  PseudoPeriodic=off  Frequencies=[]  VectorFormat=1-D array  Unit=N*m  AffineConversion=off
  PS-Simulink Converter1 : nesl_utility/PS-Simulink Converter  PhysicalDomain=network_engine_domain  SubClassName=ps_output  LeftPortType=input  RightPortType=output  PseudoPeriodic=off  Frequencies=[]  VectorFormat=1-D array  Unit=rad/s  AffineConversion=off
  Product : Product  RndMeth=Zero
  Product1 : Product  RndMeth=Zero
  Transfer Fcn (with initial outputs) : simulink_extras/Additional Linear/Transfer Fcn (with initial outputs)  N=[1]  D=[0.01 1]  Y0=HEV_Param.Control.Engine_Start_RPM  U0=HEV_Param.Control.Engine_Start_RPM
  rad/s to rpm : Constant  Value=60/(2*pi)
  Engine : PMIOPort  Side=Left
  Trans : PMIOPort  Port=2  Side=Right
  m : Outport
  tag scope: engine_speed=global
  wires:
  PS-Simulink Converter/1 -> Product1/2, Bus Creator/2  "trq"
  Product1/1 -> Bus Creator/3  "P"
  Product/1 -> [engine_speed], Transfer Fcn (with initial outputs)/1  "wEng"
  PS-Simulink Converter1/1 -> Product/1, Product1/1
  rad/s to rpm/1 -> Product/2
  Bus Creator/1 -> m/1
  Transfer Fcn (with initial outputs)/1 -> Bus Creator/1  "wEng"
  connections:
  Ideal Torque Sensor/LConn1 -- Engine/RConn1 -- Ideal Rotational Motion Sensor/LConn1
  Trans/RConn1 -- Ideal Torque Sensor/RConn1
  PS-Simulink Converter/LConn1 -- Ideal Torque Sensor/RConn2
  Ideal Rotational Motion Sensor/RConn2 -- PS-Simulink Converter1/LConn1
  Mechanical Rotational Reference/LConn1 -- Ideal Rotational Motion Sensor/RConn1

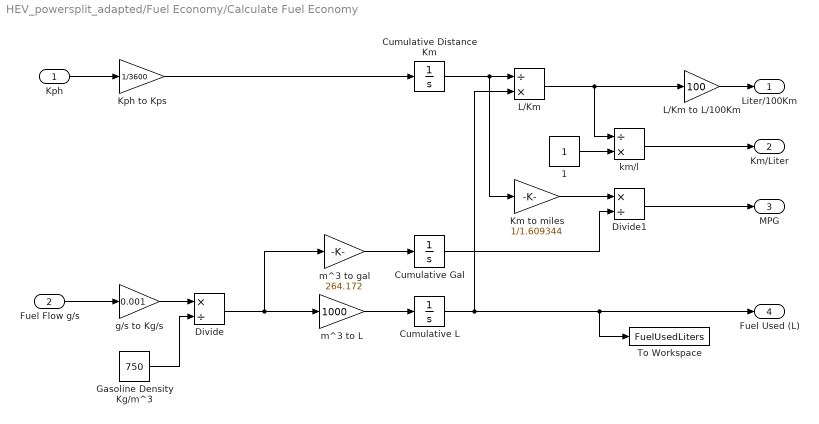
== system HEV_powersplit_adapted/Fuel Economy/Calculate Fuel Economy ==
  Kph : Inport
  Fuel Flow g/s : Inport  Port=2
  1 : Constant
  Cumulative Distance Km : Integrator  InitialCondition=eps
  Cumulative Gal : Integrator  InitialCondition=eps
  Cumulative L : Integrator  InitialCondition=eps
  Divide : Product  Inputs=*/
  Divide1 : Product  Inputs=*/
  Gasoline Density Kg/m^3 : Constant  Value=750
  Km to miles : Gain  Gain=1/1.609344
  Kph to Kps : Gain  Gain=1/3600
  L/Km : Product  Inputs=/*
  L/Km to L/100Km : Gain  Gain=100
  To Workspace : ToWorkspace  VariableName=FuelUsedLiters  SampleTime=-1
      settings: MaxDataPoints=1
  g/s to Kg/s : Gain  Gain=0.001
  km/l : Product  Inputs=/*
  m^3 to L : Gain  Gain=1000
  m^3 to gal : Gain  Gain=264.172
  Liter/100Km : Outport  VectorParamsAs1DForOutWhenUnconnected=off
  Km/Liter : Outport  Port=2  VectorParamsAs1DForOutWhenUnconnected=off
  MPG : Outport  Port=3  VectorParamsAs1DForOutWhenUnconnected=off
  Fuel Used (L) : Outport  Port=4  VectorParamsAs1DForOutWhenUnconnected=off
  wires:
  km/l/1 -> Km/Liter/1
  1/1 -> km/l/2
  Divide1/1 -> MPG/1
  L/Km to L/100Km/1 -> Liter/100Km/1
  Fuel Flow g/s/1 -> g/s to Kg/s/1
  Kph/1 -> Kph to Kps/1
  Cumulative Gal/1 -> Divide1/2
  Km to miles/1 -> Divide1/1
  L/Km/1 -> km/l/1, L/Km to L/100Km/1
  Cumulative Distance Km/1 -> Km to miles/1, L/Km/1
  Cumulative L/1 -> L/Km/2, Fuel Used (L)/1, To Workspace/1
  Kph to Kps/1 -> Cumulative Distance Km/1
  m^3 to gal/1 -> Cumulative Gal/1
  m^3 to L/1 -> Cumulative L/1
  Divide/1 -> m^3 to gal/1, m^3 to L/1
  Gasoline Density Kg/m^3/1 -> Divide/2
  g/s to Kg/s/1 -> Divide/1

== system HEV_powersplit_adapted/Kph Demand/Vehicle Speed Controller ==
  Ref Spd : Inport
  Veh Spd : Inport  Port=2
  20Hz Lowpass Filter : TransferFcn  Denominator=[1/(2*pi*20) 1]
  Accel Ctrl : Scope  NumInputPorts=4
      settings: ActiveDisplayYMinimum=-0.125  ActiveDisplayYMaximum=1.125  DataLoggingMaxPoints=100  DataLoggingDecimation=decimation  DataLoggingVariableName=ScopeData11
  Gain : Gain  Gain=200
  Ki : Gain  Gain=HEV_Param.Control.Veh_Spd.Ki
  Kp : Gain  Gain=HEV_Param.Control.Veh_Spd.Kp
  Limit Acc : Saturate  UpperLimit=1  LowerLimit=0
  Limit Brk : Saturate  UpperLimit=0  LowerLimit=-inf
  Limits [-5,5] : Integrator  LimitOutput=on  UpperSaturationLimit=5  LowerSaturationLimit=-5
  Mux : Mux  Inputs=2
  Sum : Sum  Inputs=-+|
  Sum1 : Sum  Inputs=++|
  Acc : Outport  VectorParamsAs1DForOutWhenUnconnected=off
  tag scope: BrkPedal=global
  wires:
  Limit Acc/1 -> Acc/1, Accel Ctrl/1
  Veh Spd/1 -> 20Hz Lowpass Filter/1, Mux/2
  Sum1/1 -> Limit Brk/1, Limit Acc/1, Accel Ctrl/2
  Sum/1 -> Ki/1, Kp/1, Accel Ctrl/3
  Ki/1 -> Limits [-5,5]/1
  Kp/1 -> Sum1/2
  Limits [-5,5]/1 -> Sum1/1
  20Hz Lowpass Filter/1 -> Sum/1
  Mux/1 -> Accel Ctrl/4
  Limit Brk/1 -> Gain/1
  Gain/1 -> [BrkPedal]
  Ref Spd/1 -> Sum/2, Mux/1
